simulink library "STMM"  (R2024a)
settings: Solver=VariableStepAuto  StartTime=0.0  StopTime=10.0  RelTol=1e-3
undefined symbols (not defined in the file or in its folder): raptor_xcp_function, StateCAN
libraries: Utilities x260, Raptor_lib x68, simulink x2
(part 1 of 3)
settings Model: Creator=serga  LastModifiedBy=serga

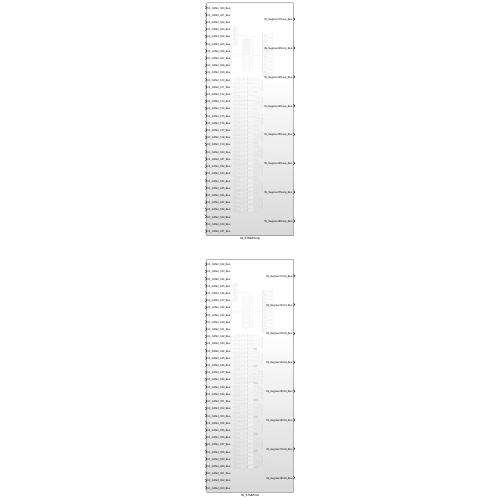
[thumbnail: Simulink's stored preview of the top-level diagram]
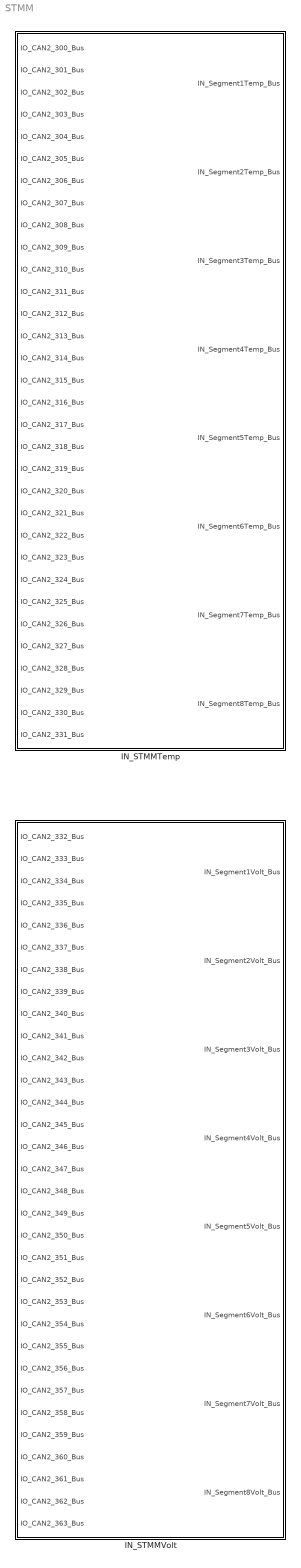
== system STMM ==
  IN_STMMTemp : Subsystem
  IN_STMMVolt : Subsystem
